simulink model "per_char"  (R2017b)
settings: Solver=VariableStepAuto  StartTime=0.0  StopTime=10.0  RelTol=1e-3
settings Model: Creator=foton  LastModifiedBy=foton

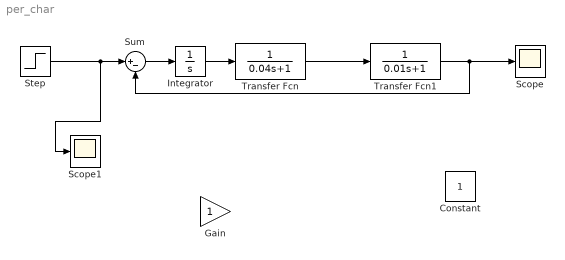
== system per_char ==
  Constant : Constant
  Gain : Gain
  Integrator : Integrator
  Scope : Scope
  Scope1 : Scope
  Step : Step  Time=0  Before=1  SampleTime=0
  Sum : Sum  Inputs=|+-
  Transfer Fcn : TransferFcn  Denominator=[0.04 1]
  Transfer Fcn1 : TransferFcn  Denominator=[0.01 1]
  wires:
  Step/1 -> Sum/1, Scope1/1
  Transfer Fcn/1 -> Transfer Fcn1/1
  Integrator/1 -> Transfer Fcn/1
  Transfer Fcn1/1 -> Sum/2, Scope/1
  Sum/1 -> Integrator/1
